simulink model "TP4"  (Simulink 7.4)
settings: Solver=ode45  StartTime=0.0  StopTime=1000  RelTol=1e-3
PreLoadFcn:
  | mamdani_25_gauss_minmax_centroid = readfis('mamdani_25_gauss_minmax_centroid');
  | mamdani_25_gauss_minmax_medmax = readfis('mamdani_25_gauss_minmax_medmax');
  | mamdani_25_gauss_prod_centroide = readfis('mamdani_25_gauss_prod_centroide');
  | mamdani_25_gauss_prod_medmax = readfis('mamdani_25_gauss_prod_medmax');
  | mamdani_25_trimf_minmax_centroide = readfis('mamdani_25_trimf_minmax_centroide');
  | mamdani_25_trimf_minmax_medmax = readfis('mamdani_25_trimf_minmax_medmax');
  | mamdani_25_trimf_prod_centroide = readfis('mamdani_25_trimf_prod_centroide');
  | mamdani_25_trimf_prod_medmax = readfis('mamdani_25_trimf_prod_medmax');
  | mamdani_9_gaussmf_minmax_centoide = readfis('mamdani_9_gaussmf_minmax_centoide');
  | mamdani_9_gaussmf_minmax_medmax = readfis('mamdani_9_gaussmf_minmax_medmax');
  | mamdani_9_gaussmf_prod_centroide = readfis('mamdani_9_gaussmf_prod_centroide');
  | mamdani_9_gaussmf_prod_medmax = readfis('mamdani_9_gaussmf_prod_medmax');
  | mamdani_9_trimf_minmax_centroide = readfis('mamdani_9_trimf_minmax_centroide');
  | mamdani_9_trimf_minmax_medmax = readfis('mamdani_9_trimf_minmax_medmax');
  | mamdani_9_trimf_prod_centroide = readfis('mamdani_9_trimf_prod_centroide');
  | mamdani_9_trimf_prod_medmax = readfis('mamdani_9_trimf_prod_medmax');
  | sugeno_25_gausmf_minmax_med = readfis('sugeno_25_gausmf_minmax_med');
  | sugeno_25_gausmf_minmax_sum = readfis('sugeno_25_gausmf_minmax_sum');
  | sugeno_25_gausmf_prod_med = readfis('sugeno_25_gausmf_prod_med');
  | sugeno_25_gausmf_prod_sum = readfis('sugeno_25_gausmf_prod_sum');
  | sugeno_25_trimf_minmax_med = readfis('sugeno_25_trimf_minmax_med');
  | sugeno_25_trimf_minmax_sum = readfis('sugeno_25_trimf_minmax_sum');
  | sugeno_25_trimf_prod_med = readfis('sugeno_25_trimf_prod_med');
  | sugeno_25_trimf_prod_sum = readfis('sugeno_25_trimf_prod_sum');
  | sugeno_9_gaussmf_minmax_med = readfis('sugeno_9_gaussmf_minmax_med');
  | sugeno_9_gaussmf_minmax_sum = readfis('sugeno_9_gaussmf_minmax_sum');
  | sugeno_9_gaussmf_prod_med = readfis('sugeno_9_gaussmf_prod_med');
  | sugeno_9_gaussmf_prod_sum = readfis('sugeno_9_gaussmf_prod_sum');
  | sugeno_9_trimf_minmax_med = readfis('sugeno_9_trimf_minmax_med');
  | sugeno_9_trimf_minmax_sum = readfis('sugeno_9_trimf_minmax_sum');
  | sugeno_9_trimf_prod_med   = readfis('sugeno_9_trimf_prod_med');
  | sugeno_9_trimf_prod_sum = readfis('sugeno_9_trimf_prod_sum');
libraries: fuzblock x3
settings Model: Creator=Sergio  LastModifiedBy=Sergio
settings SolverCC: ZeroCrossControl=DisableAll  ZeroCrossAlgorithm=Adaptive

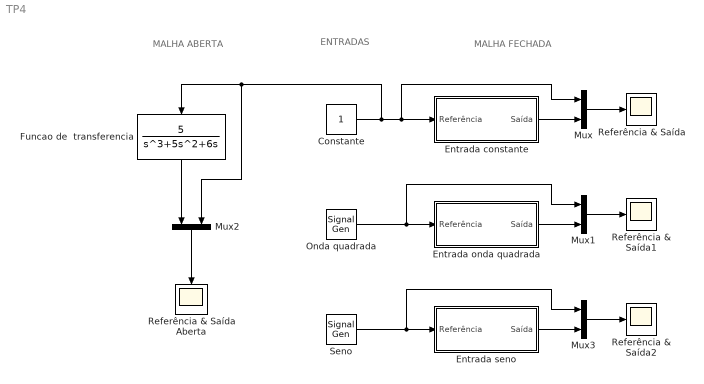
== system TP4 ==
  note: ENTRADAS
  note: MALHA ABERTA
  note: MALHA FECHADA
  Constante : Constant  OutDataType=fixdt(1, 16)  OutScaling=2^0
  Entrada constante : Subsystem  mask{controllerType=sugeno_25_trimf_minmax_sum, factorEscala1=1, factorEscala2=5}
      mask prompts: controllerType "Fuzzy Controller Type"; factorEscala1 "Factor Escala 1"; factorEscala2 "Factor Escala 2"
      mask StyleString: popup(mamdani_25_gauss_minmax_centroid|mamdani_25_gauss_minmax_medmax|mamdani_25_gauss_prod_centroide|mamdani_25_gauss_prod_medmax|mamdani_25_trimf_minmax_centroide|mamdani_25_trimf_minmax_medmax|mamdani_25_trimf_prod_centroide|mamdani_25_trimf_prod_medmax|mamdani_9_gaussmf_minmax_centoide|mamdani_9_gaussmf_minmax_medmax|mamdani_9_gaussmf_prod_centroide|mamdani_9_gaussmf_prod_medmax|mamdani_9_trimf_minmax_centroide|mamdani_9_trimf_minmax_medmax|mamdani_9_trimf_prod_centroide|mamdani_9_trimf_prod_medmax|sugeno_25_gausmf_minmax_med   |sugeno_25_gausmf_minmax_sum|sugeno_25_gausmf_prod_med|sugeno_25_gausmf_prod_sum|sugeno_25_trimf_minmax_med|sugeno_25_trimf_minmax_sum|sugeno_25_trimf_prod_med|sugeno_25_trimf_prod_sum|sugeno_9_gaussmf_minmax_med|sugeno_9_gaussmf_minmax_sum|sugeno_9_gaussmf_prod_med|sugeno_9_gaussmf_prod_sum|sugeno_9_trimf_minmax_med|sugeno_9_trimf_minmax_sum|sugeno_9_trimf_prod_med  |sugeno_9_trimf_prod_sum),edit,edit
      mask CallbackString:
      | t = char(get_param(gcb,'controllerType'));
      | set_param(char(find_system(gcb,'LookUnderMasks','all','Tag','controller')),'fismatrix',t);|f = char(get_param(gcb,'factorEscala1'));
      | set_param(char(find_system(gcb,'LookUnderMasks','all','Tag','factor1')),'gain',f);|f = char(get_param(gcb,'factorEscala2'));
      | set_param(char(find_system(gcb,'LookUnderMasks','all','Tag','factor2')),'gain',f);
  Entrada onda quadrada : Subsystem  mask{controllerType=sugeno_25_trimf_minmax_sum, factorEscala1=0.1, factorEscala2=5}
      mask prompts: controllerType "Fuzzy Controller Type"; factorEscala1 "Factor Escala 1"; factorEscala2 "Factor Escala 2"
      mask StyleString: popup(mamdani_25_gauss_minmax_centroid|mamdani_25_gauss_minmax_medmax|mamdani_25_gauss_prod_centroide|mamdani_25_gauss_prod_medmax|mamdani_25_trimf_minmax_centroide|mamdani_25_trimf_minmax_medmax|mamdani_25_trimf_prod_centroide|mamdani_25_trimf_prod_medmax|mamdani_9_gaussmf_minmax_centoide|mamdani_9_gaussmf_minmax_medmax|mamdani_9_gaussmf_prod_centroide|mamdani_9_gaussmf_prod_medmax|mamdani_9_trimf_minmax_centroide|mamdani_9_trimf_minmax_medmax|mamdani_9_trimf_prod_centroide|mamdani_9_trimf_prod_medmax|sugeno_25_gausmf_minmax_med   |sugeno_25_gausmf_minmax_sum|sugeno_25_gausmf_prod_med|sugeno_25_gausmf_prod_sum|sugeno_25_trimf_minmax_med|sugeno_25_trimf_minmax_sum|sugeno_25_trimf_prod_med|sugeno_25_trimf_prod_sum|sugeno_9_gaussmf_minmax_med|sugeno_9_gaussmf_minmax_sum|sugeno_9_gaussmf_prod_med|sugeno_9_gaussmf_prod_sum|sugeno_9_trimf_minmax_med|sugeno_9_trimf_minmax_sum|sugeno_9_trimf_prod_med  |sugeno_9_trimf_prod_sum),edit,edit
      mask CallbackString:
      | t = char(get_param(gcb,'controllerType'));
      | set_param(char(find_system(gcb,'LookUnderMasks','all','Tag','controller')),'fismatrix',t);|f = char(get_param(gcb,'factorEscala1'));
      | set_param(char(find_system(gcb,'LookUnderMasks','all','Tag','factor1')),'gain',f);|f = char(get_param(gcb,'factorEscala2'));
      | set_param(char(find_system(gcb,'LookUnderMasks','all','Tag','factor2')),'gain',f);
  Entrada seno : Subsystem  mask{controllerType=sugeno_25_trimf_minmax_sum, factorEscala1=5, factorEscala2=5}
      mask prompts: controllerType "Fuzzy Controller Type"; factorEscala1 "Factor Escala 1"; factorEscala2 "Factor Escala 2"
      mask StyleString: popup(mamdani_25_gauss_minmax_centroid|mamdani_25_gauss_minmax_medmax|mamdani_25_gauss_prod_centroide|mamdani_25_gauss_prod_medmax|mamdani_25_trimf_minmax_centroide|mamdani_25_trimf_minmax_medmax|mamdani_25_trimf_prod_centroide|mamdani_25_trimf_prod_medmax|mamdani_9_gaussmf_minmax_centoide|mamdani_9_gaussmf_minmax_medmax|mamdani_9_gaussmf_prod_centroide|mamdani_9_gaussmf_prod_medmax|mamdani_9_trimf_minmax_centroide|mamdani_9_trimf_minmax_medmax|mamdani_9_trimf_prod_centroide|mamdani_9_trimf_prod_medmax|sugeno_25_gausmf_minmax_med   |sugeno_25_gausmf_minmax_sum|sugeno_25_gausmf_prod_med|sugeno_25_gausmf_prod_sum|sugeno_25_trimf_minmax_med|sugeno_25_trimf_minmax_sum|sugeno_25_trimf_prod_med|sugeno_25_trimf_prod_sum|sugeno_9_gaussmf_minmax_med|sugeno_9_gaussmf_minmax_sum|sugeno_9_gaussmf_prod_med|sugeno_9_gaussmf_prod_sum|sugeno_9_trimf_minmax_med|sugeno_9_trimf_minmax_sum|sugeno_9_trimf_prod_med  |sugeno_9_trimf_prod_sum),edit,edit
      mask CallbackString:
      | t = char(get_param(gcb,'controllerType'));
      | set_param(char(find_system(gcb,'LookUnderMasks','all','Tag','controller')),'fismatrix',t);|f = char(get_param(gcb,'factorEscala1'));
      | set_param(char(find_system(gcb,'LookUnderMasks','all','Tag','factor1')),'gain',f);|f = char(get_param(gcb,'factorEscala2'));
      | set_param(char(find_system(gcb,'LookUnderMasks','all','Tag','factor2')),'gain',f);
  Funcao de  transferencia : TransferFcn  Numerator=[5]  Denominator=[1 5 6 0]
  Mux{,1..3} (4 alike) : Mux  Inputs=2
  Onda quadrada : SignalGenerator  WaveForm=square  Frequency=0.01
  Referência & Saída : Scope
      settings: YMin=1  YMax=1
  Referência & Saída Aberta : Scope
      settings: YMin=0  YMax=20  SaveName=ScopeData3
  Referência & Saída1 : Scope
      settings: YMin=-1  YMax=1  SaveName=ScopeData4
  Referência & Saída2 : Scope
      settings: YMin=-1.1  YMax=1.1  SaveName=ScopeData5
  Seno : SignalGenerator  Frequency=0.01
  wires:
  Entrada constante/1(Saída) -> Mux/2
  Mux/1 -> Referência & Saída/1
  Mux2/1 -> Referência & Saída Aberta/1
  Entrada onda quadrada/1(Saída) -> Mux1/2
  Mux1/1 -> Referência & Saída1/1
  Entrada seno/1(Saída) -> Mux3/2
  Mux3/1 -> Referência & Saída2/1
  Constante/1 -> Mux/1, Entrada constante/1(Referência), Funcao de  transferencia/1, Mux2/2
  Onda quadrada/1 -> Mux1/1, Entrada onda quadrada/1(Referência)
  Seno/1 -> Mux3/1, Entrada seno/1(Referência)
  Funcao de  transferencia/1 -> Mux2/1

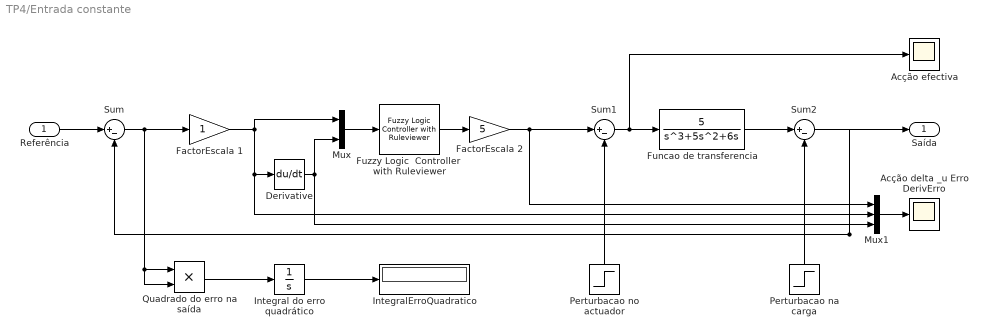
== system TP4/Entrada constante ==
  Referência : Inport  OutDataType=fixdt(1, 16)  OutScaling=2^0
  Acção delta _u Erro DerivErro : Scope
      settings: YMin=0  YMax=3.75e-005  SaveName=ScopeData2
  Acção efectiva : Scope
      settings: YMin=-1.5  YMax=1.25
  Derivative : Derivative
  FactorEscala 1 : Gain  Tag=factor1  ParameterDataType=fixdt(1, 16)  ParameterScaling=2^0  OutDataType=fixdt(1, 16)  OutScaling=2^0
  FactorEscala 2 : Gain  Tag=factor2  Gain=5  ParameterDataType=fixdt(1, 16)  ParameterScaling=2^0  OutDataType=fixdt(1, 16)  OutScaling=2^0
  Funcao de transferencia : TransferFcn  Numerator=[5]  Denominator=[1 5 6 0]
  Fuzzy Logic  Controller  with Ruleviewer : fuzblock/Fuzzy Logic  Controller  with Ruleviewer  Tag=controller  SystemSampleTime=-1  fismatrix=sugeno_25_trimf_minmax_sum  Ts=2
  Integral do erro quadrático : Integrator
  IntegralErroQuadratico : Display
  Mux : Mux  Inputs=2
  Mux1 : Mux  Inputs=3
  Perturbacao na carga : Step  Time=200  After=0.1  SampleTime=0
  Perturbacao no actuador : Step  Time=200  After=0.1  SampleTime=0
  Quadrado do erro na saída : Product  OutDataType=fixdt(1, 16)  OutScaling=2^0  RndMeth=Zero
  Sum : Sum  Inputs=|+-  OutDataType=fixdt(1, 16)  OutScaling=2^0
  Sum1 : Sum  Inputs=|+-  OutDataType=fixdt(1, 16)  OutScaling=2^0
  Sum2 : Sum  Inputs=|+-  OutDataType=fixdt(1, 16)  OutScaling=2^0
  Saída : Outport  OutDataType=fixdt(1, 16)  OutScaling=2^0
  wires:
  Referência/1 -> Sum/1
  Sum/1 -> FactorEscala 1/1, Quadrado do erro na saída/1, Quadrado do erro na saída/2
  Quadrado do erro na saída/1 -> Integral do erro quadrático/1
  Integral do erro quadrático/1 -> IntegralErroQuadratico/1
  FactorEscala 1/1 -> Mux/1, Mux1/2, Derivative/1
  Mux1/1 -> Acção delta _u Erro DerivErro/1
  Mux/1 -> Fuzzy Logic  Controller  with Ruleviewer/1
  Fuzzy Logic  Controller  with Ruleviewer/1 -> FactorEscala 2/1
  Derivative/1 -> Mux/2, Mux1/3
  Sum2/1 -> Saída/1, Sum/2
  FactorEscala 2/1 -> Mux1/1, Sum1/1
  Sum1/1 -> Funcao de transferencia/1, Acção efectiva/1
  Funcao de transferencia/1 -> Sum2/1
  Perturbacao no actuador/1 -> Sum1/2
  Perturbacao na carga/1 -> Sum2/2

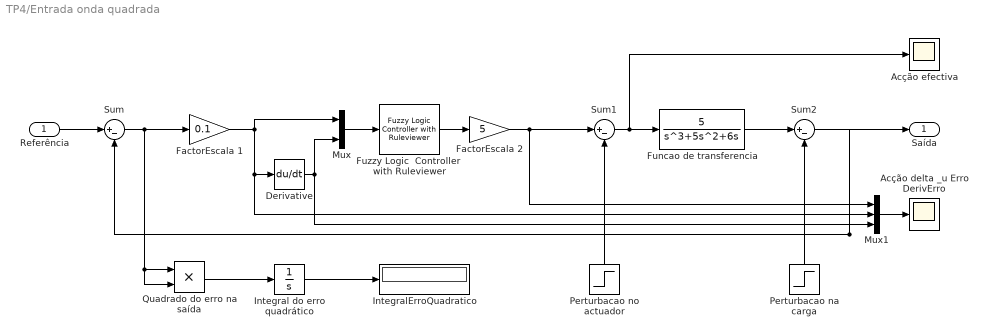
== system TP4/Entrada onda quadrada ==
  Referência : Inport  OutDataType=fixdt(1, 16)  OutScaling=2^0
  Acção delta _u Erro DerivErro : Scope
      settings: YMin=0  YMax=3.75e-005  SaveName=ScopeData2
  Acção efectiva : Scope
      settings: YMin=-1.5  YMax=1.25
  Derivative : Derivative
  FactorEscala 1 : Gain  Tag=factor1  Gain=0.1  ParameterDataType=fixdt(1, 16)  ParameterScaling=2^0  OutDataType=fixdt(1, 16)  OutScaling=2^0
  FactorEscala 2 : Gain  Tag=factor2  Gain=5  ParameterDataType=fixdt(1, 16)  ParameterScaling=2^0  OutDataType=fixdt(1, 16)  OutScaling=2^0
  Funcao de transferencia : TransferFcn  Numerator=[5]  Denominator=[1 5 6 0]
  Fuzzy Logic  Controller  with Ruleviewer : fuzblock/Fuzzy Logic  Controller  with Ruleviewer  Tag=controller  SystemSampleTime=-1  fismatrix=sugeno_25_trimf_minmax_sum  Ts=2
  Integral do erro quadrático : Integrator
  IntegralErroQuadratico : Display
  Mux : Mux  Inputs=2
  Mux1 : Mux  Inputs=3
  Perturbacao na carga : Step  Time=200  After=0  SampleTime=0
  Perturbacao no actuador : Step  Time=100  After=0  SampleTime=0
  Quadrado do erro na saída : Product  OutDataType=fixdt(1, 16)  OutScaling=2^0  RndMeth=Zero
  Sum : Sum  Inputs=|+-  OutDataType=fixdt(1, 16)  OutScaling=2^0
  Sum1 : Sum  Inputs=|+-  OutDataType=fixdt(1, 16)  OutScaling=2^0
  Sum2 : Sum  Inputs=|+-  OutDataType=fixdt(1, 16)  OutScaling=2^0
  Saída : Outport  OutDataType=fixdt(1, 16)  OutScaling=2^0
  wires:
  Referência/1 -> Sum/1
  Sum/1 -> FactorEscala 1/1, Quadrado do erro na saída/1, Quadrado do erro na saída/2
  Quadrado do erro na saída/1 -> Integral do erro quadrático/1
  Integral do erro quadrático/1 -> IntegralErroQuadratico/1
  FactorEscala 1/1 -> Mux/1, Mux1/2, Derivative/1
  Mux1/1 -> Acção delta _u Erro DerivErro/1
  Mux/1 -> Fuzzy Logic  Controller  with Ruleviewer/1
  Fuzzy Logic  Controller  with Ruleviewer/1 -> FactorEscala 2/1
  Derivative/1 -> Mux/2, Mux1/3
  Sum2/1 -> Saída/1, Sum/2
  FactorEscala 2/1 -> Mux1/1, Sum1/1
  Sum1/1 -> Funcao de transferencia/1, Acção efectiva/1
  Funcao de transferencia/1 -> Sum2/1
  Perturbacao no actuador/1 -> Sum1/2
  Perturbacao na carga/1 -> Sum2/2

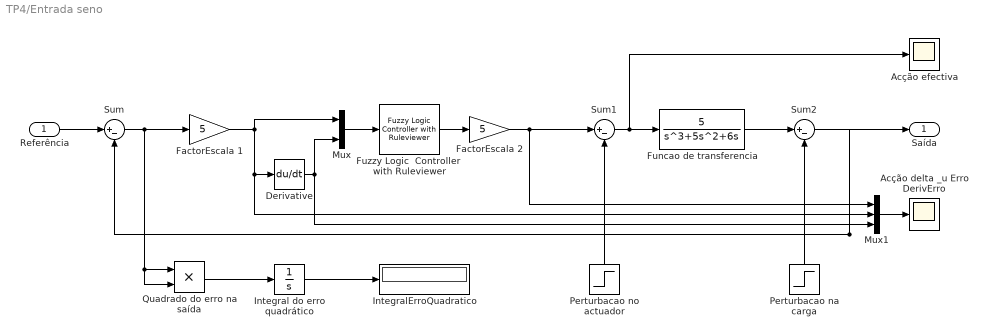
== system TP4/Entrada seno ==
  Referência : Inport  OutDataType=fixdt(1, 16)  OutScaling=2^0
  Acção delta _u Erro DerivErro : Scope
      settings: YMin=0  YMax=3.75e-005  SaveName=ScopeData2
  Acção efectiva : Scope
      settings: YMin=-1.5  YMax=1.25
  Derivative : Derivative
  FactorEscala 1 : Gain  Tag=factor1  Gain=5  ParameterDataType=fixdt(1, 16)  ParameterScaling=2^0  OutDataType=fixdt(1, 16)  OutScaling=2^0
  FactorEscala 2 : Gain  Tag=factor2  Gain=5  ParameterDataType=fixdt(1, 16)  ParameterScaling=2^0  OutDataType=fixdt(1, 16)  OutScaling=2^0
  Funcao de transferencia : TransferFcn  Numerator=[5]  Denominator=[1 5 6 0]
  Fuzzy Logic  Controller  with Ruleviewer : fuzblock/Fuzzy Logic  Controller  with Ruleviewer  Tag=controller  SystemSampleTime=-1  fismatrix=sugeno_25_trimf_minmax_sum  Ts=2
  Integral do erro quadrático : Integrator
  IntegralErroQuadratico : Display
  Mux : Mux  Inputs=2
  Mux1 : Mux  Inputs=3
  Perturbacao na carga : Step  Time=200  After=0  SampleTime=0
  Perturbacao no actuador : Step  Time=100  After=0  SampleTime=0
  Quadrado do erro na saída : Product  OutDataType=fixdt(1, 16)  OutScaling=2^0  RndMeth=Zero
  Sum : Sum  Inputs=|+-  OutDataType=fixdt(1, 16)  OutScaling=2^0
  Sum1 : Sum  Inputs=|+-  OutDataType=fixdt(1, 16)  OutScaling=2^0
  Sum2 : Sum  Inputs=|+-  OutDataType=fixdt(1, 16)  OutScaling=2^0
  Saída : Outport  OutDataType=fixdt(1, 16)  OutScaling=2^0
  wires:
  Referência/1 -> Sum/1
  Sum/1 -> FactorEscala 1/1, Quadrado do erro na saída/1, Quadrado do erro na saída/2
  Quadrado do erro na saída/1 -> Integral do erro quadrático/1
  Integral do erro quadrático/1 -> IntegralErroQuadratico/1
  FactorEscala 1/1 -> Mux/1, Mux1/2, Derivative/1
  Mux1/1 -> Acção delta _u Erro DerivErro/1
  Mux/1 -> Fuzzy Logic  Controller  with Ruleviewer/1
  Fuzzy Logic  Controller  with Ruleviewer/1 -> FactorEscala 2/1
  Derivative/1 -> Mux/2, Mux1/3
  Sum2/1 -> Saída/1, Sum/2
  FactorEscala 2/1 -> Mux1/1, Sum1/1
  Sum1/1 -> Funcao de transferencia/1, Acção efectiva/1
  Funcao de transferencia/1 -> Sum2/1
  Perturbacao no actuador/1 -> Sum1/2
  Perturbacao na carga/1 -> Sum2/2
